simulink model "pdf_subsis1"  (R2023a)
settings: Solver=VariableStepAuto  StartTime=0.0  StopTime=10.0  RelTol=1e-3
values from neighbouring files (symbols this model uses):
  Ks_range = zeros(2,5*size(Vs_range,2))    [PI_6_Tracker_bigGuy.m]
  Vs_range = [10; 45]    [PI_6_Tracker_bigGuy.m]
settings Model: Creator=ignac  LastModifiedBy=ignac

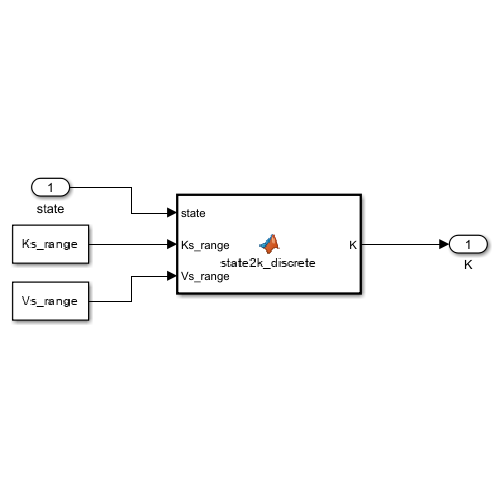
[thumbnail: Simulink's stored preview of the top-level diagram]
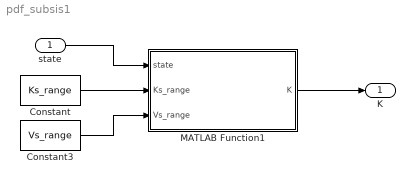
== system pdf_subsis1 ==
  state : Inport
  Constant : Constant  Value=Ks_range
  Constant3 : Constant  Value=Vs_range
  MATLAB Function1 : MATLAB Function  TreatAsAtomicUnit=on
  K : Outport
  wires:
  Constant/1 -> MATLAB Function1/2(Ks_range)
  state/1 -> MATLAB Function1/1(state)
  MATLAB Function1/1(K) -> K/1
  Constant3/1 -> MATLAB Function1/3(Vs_range)

== matlab function pdf_subsis1/MATLAB Function1 ==
  data: state input; K output; Ks_range input; Vs_range input
function K = state2k_discrete(state, Ks_range, Vs_range)
    % state = [V, H] instantánea
    % Ks_range = [K1, K2, K3, ...], con sus dimensiones (2,5,[])
    % Vs_range = [[V_start1;V_end1], [V_start2;V_end2],...]
    % El rango de V en el que va el controlador K3 es entre Vs_range(1,3) y
    % Vs_range(2,3).
    % K2 se usa entre [V_start2, V_end2).
    % Ejemplo: Para tener un controlador K1 entre 10 y 15 m/s, otro K2 entre
    % los 15 y los 20, otro K3 entre 20 y 25 y K4 entre 25 y 30 m/s, argumentos:
    % Ks_range = [K1, K2, K3, K4]
    % Vs_range = [[10; 15], [15;20], [20;25], [25;30]];
    
    V = state(1);
    % H = state(2);

    K = zeros(2,5);

    Ks = reshape(Ks_range,2,5,[]);
    found = 0;

    for i = 1:size(Vs_range,2)
        range = Vs_range(:,i);
        if V >= range(1) && V < range(2)
            K = Ks(:,:,i);
            found = 1;
            disp(i)
        end
    end

    if ~found
        K = zeros(2,5);
        disp('ERROR: state2k_discrete: Range not satisfied.')
    end
end
